simulink model "assignment_6"  (R2020b)
settings: Solver=VariableStepAuto  StartTime=0.0  StopTime=10.0  RelTol=1e-3
settings Model: Creator=Sudhanshu  LastModifiedBy=Sudhanshu

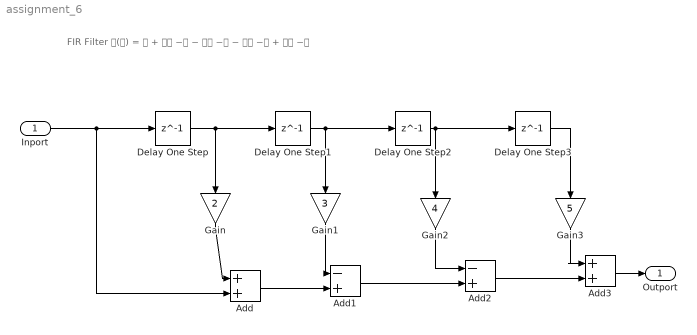
== system assignment_6 ==
  note: FIR Filter
      | 𝐇(𝐳) = 𝟏 + 𝟐𝐳 −𝟏 − 𝟑𝐳 −𝟐 − 𝟒𝐳 −𝟑 + 𝟓𝐳 −𝟒
  Inport : Inport
  Add : Sum
  Add1 : Sum  Inputs=-+
  Add2 : Sum  Inputs=-+
  Add3 : Sum
  Delay One Step{,1..3} (4 alike) : Delay  DelayLength=1
  Gain : Gain  Gain=2
  Gain1 : Gain  Gain=3
  Gain2 : Gain  Gain=4
  Gain3 : Gain  Gain=5
  Outport : Outport
  wires:
  Inport/1 -> Add/2, Delay One Step/1
  Add2/1 -> Add3/2
  Add1/1 -> Add2/2
  Add/1 -> Add1/2
  Delay One Step/1 -> Gain/1, Delay One Step1/1
  Delay One Step1/1 -> Gain1/1, Delay One Step2/1
  Delay One Step2/1 -> Gain2/1, Delay One Step3/1
  Delay One Step3/1 -> Gain3/1
  Gain3/1 -> Add3/1
  Gain2/1 -> Add2/1
  Gain1/1 -> Add1/1
  Gain/1 -> Add/1
  Add3/1 -> Outport/1
